simulink model "six_plus_six_AcmsteeringV09_main_1lf"  (R2014a)
settings: Solver=FixedStepDiscrete  StartTime=0.0  StopTime=10.0  FixedStep=0.0005  RelTol=1e-3
InitFcn:
  | Veh_Par_wxt
undefined symbols (not defined in the file or in its folder): acc_spdctl, ag_thr, B, bra_em, bra_pre_gz2, bra_pre_gz34, bra_pre_yd, brakepre_dem_data, brakeTrq_dem_data, bratrq_max, ecucoder_acal, eff_tran, ESP_switch, G, guzhang_lf, guzhang_lm, guzhang_lr, guzhang_rf, guzhang_rm, guzhang_rr, kd1, kd2, ki1, ki2, kp1, kp2, L, myFIS, premax, Radius, RC_switch, s_opt_yi, s_opt_zhuan, s_opt_zhuan_add, s_opt_zhuan_table, spd_map_mot, spd_spdctl, speed_thr_park, TCS_switch, tras_ratio, trq_map_mot, trqmax_yd, trqmax_zx, trqmaxneg, v_gain, v_table, v_thr_park, zhidong_bianmazhi, zhidong_down, zhidong_up, zhidong_youmen, zhuanxiang_bianmazhi, zhuanxiang_down, zhuanxiang_up, zhuanxiang_youmen
libraries: simulink x980, ec5744lib x59, fuzblock x2
(part 8 of 25)

== matlab function six_plus_six_AcmsteeringV09_main_1lf/MainControl/mode_control/center_steer/center_steer/容错控制/MATLAB Function ==
  data: trq_dem_l input; trq_dem_lf output; trq_dem_lm output; trq_dem_r input; trqlim_lf input; trqlim_lm input; trqlim_lr input; trqlim_rf input; trqlim_rm input; trqlim_rr input; guzhang_lf input; guzhang_lm input; guzhang_lr input; guzhang_rf input; guzhang_rm input; guzhang_rr input; trq_dem_lr output; trq_dem_rf output; trq_dem_rm output; trq_dem_rr output; bra_pre_l output; bra_pre_r output; bra_pre_yd input; mode output; bra_dem_l input; bra_dem_r input; brake_dem input
function [trq_dem_lf,trq_dem_lm,trq_dem_lr,trq_dem_rf,trq_dem_rm,trq_dem_rr,bra_pre_l,bra_pre_r,mode] = fcn(trq_dem_l,trq_dem_r,trqlim_lf,trqlim_lm,trqlim_lr,trqlim_rf,trqlim_rm,trqlim_rr,guzhang_lf,guzhang_lm,guzhang_lr,guzhang_rf,guzhang_rm,guzhang_rr,bra_pre_yd,bra_dem_l,bra_dem_r,brake_dem)
%#codegen
if brake_dem==0
    
    trq_dem_lf=single(trq_dem_l/3);
    trq_dem_lm=single(trq_dem_l/3);
    trq_dem_lr=single(trq_dem_l/3);
    trq_dem_rf=single(trq_dem_r/3);
    trq_dem_rm=single(trq_dem_r/3);
    trq_dem_rr=single(trq_dem_r/3);
    bra_pre_l=single(0);
    bra_pre_r=single(0);
    mode=1;
    
    
    %     if guzhang_lf==0 && guzhang_lr==0 && guzhang_rf==0 && guzhang_rr==0    %0电机故障,平均分配
    %         trq_dem_lf=single(trq_dem_l/2);
    %         trq_dem_lr=single(trq_dem_l/2);
    %         trq_dem_rf=single(trq_dem_r/2);
    %         trq_dem_rr=single(trq_dem_r/2);
    %         bra_pre_l=single(0);
    %         bra_pre_r=single(0);
    %         mode=1;
    %     elseif  guzhang_lf==1 && guzhang_lr==0 && guzhang_rf==0 && guzhang_rr==0  %1电机故障，同侧电机进行力矩转移,跟行车不同，对侧不降扭。
    %         trq_dem_lf=single(0);
    %         trq_dem_lr=single(min(trq_dem_l,trqlim_lr));
    %         trq_dem_rf=single(trq_dem_r/2);
    %         trq_dem_rr=single(trq_dem_r/2);
    %         bra_pre_l=single(0);
    %         bra_pre_r=single(0);
    %         mode=2;
    %     elseif  guzhang_lf==0 && guzhang_lr==1 && guzhang_rf==0 && guzhang_rr==0
    %         trq_dem_lf=single(min(trq_dem_l,trqlim_lf));
    %         trq_dem_lr=single(0);
    %         trq_dem_rf=single(trq_dem_r/2);
    %         trq_dem_rr=single(trq_dem_r/2);
    %         bra_pre_l=single(0);
    %         bra_pre_r=single(0);
    %         mode=3;
    %     elseif  guzhang_lf==0 && guzhang_lr==0 && guzhang_rf==1 && guzhang_rr==0
    %         trq_dem_rf=single(0);
    %         trq_dem_rr=single(min(trq_dem_r,trqlim_rr));
    %         trq_dem_lf=single(trq_dem_l/2);
    %         trq_dem_lr=single(trq_dem_l/2);
    %         bra_pre_l=single(0);
    %         bra_pre_r=single(0);
    %         mode=4;
    %     elseif  guzhang_lf==0 && guzhang_lr==0 && guzhang_rf==0 && guzhang_rr==1
    %         trq_dem_rf=single(min(trq_dem_r,trqlim_rf));
    %         trq_dem_rr=single(0);
    %         trq_dem_lf=single(trq_dem_l/2);
    %         trq_dem_lr=single(trq_dem_l/2);
    %         bra_pre_l=single(0);
    %         bra_pre_r=single(0);
    %         mode=5;
    %     elseif  guzhang_lf==1 && guzhang_lr==1 && guzhang_rf==0 && guzhang_rr==0  %2电机故障，左侧双电机故障，左侧履带施加制动，改为原地转向
    %         trq_dem_lf=single(0);
    %         trq_dem_lr=single(0);
    %         trq_dem_rf=single(trq_dem_r/2);
    %         trq_dem_rr=single(trq_dem_r/2);
    %         bra_pre_l=single(bra_pre_yd);
    %         bra_pre_r=single(0);
    %         mode=6;
    %     elseif  guzhang_lf==0 && guzhang_lr==0 && guzhang_rf==1 && guzhang_rr==1  %右侧双电机故障
    %         trq_dem_lf=single(trq_dem_l/2);
    %         trq_dem_lr=single(trq_dem_l/2);
    %         trq_dem_rf=single(0);
    %         trq_dem_rr=single(0);
    %         bra_pre_l=single(0);
    %         bra_pre_r=single(bra_pre_yd);
    %         mode=7;
    %     elseif  guzhang_lf==1 && guzhang_lr==0 && guzhang_rf==1 && guzhang_rr==0 %2电机故障，对侧双电机故障,有4种情况,前两电机故障
    %         trq_dem_lf=single(0);
    %         trq_dem_rf=single(0);
    %         trq_dem_lr=single(min(trq_dem_l,trqlim_lr));
    %         trq_dem_rr=single(min(trq_dem_r,trqlim_rr));
    %         bra_pre_l=single(0);
    %         bra_pre_r=single(0);
    %         mode=8;
    %     elseif  guzhang_lf==0 && guzhang_lr==1 && guzhang_rf==0 && guzhang_rr==1 %后两电机故障
    %         trq_dem_lr=single(0);
    %         trq_dem_rr=single(0);
    %         trq_dem_lf=single(min(trq_dem_l,trqlim_lf));
    %         trq_dem_rf=single(min(trq_dem_r,trqlim_rf));
    %         bra_pre_l=single(0);
    %         bra_pre_r=single(0);
    %         mode=9;
    %     elseif  guzhang_lf==1 && guzhang_lr==0 && guzhang_rf==0 && guzhang_rr==1 %左前电机和右后电机故障
    %         trq_dem_lf=single(0);
    %         trq_dem_rr=single(0);
    %         trq_dem_lr=single(min(trq_dem_l,trqlim_lr));
    %         trq_dem_rf=single(min(trq_dem_r,trqlim_rf));
    %         bra_pre_l=single(0);
    %         bra_pre_r=single(0);
    %         mode=10;
    %     elseif  guzhang_lf==0 && guzhang_lr==1 && guzhang_rf==1 && guzhang_rr==0 %左后电机和右前电机故障
    %         trq_dem_lr=single(0);
    %         trq_dem_rf=single(0);
    %         trq_dem_lf=single(min(trq_dem_l,trqlim_lf));
    %         trq_dem_rr=single(min(trq_dem_r,trqlim_rr));
    %         bra_pre_l=single(0);
    %         bra_pre_r=single(0);
    %         mode=11;
    %     elseif guzhang_lf==1 && guzhang_lr==1 && guzhang_rf==1 && guzhang_rr==0   % 三电机故障
    %         trq_dem_lf=single(0);
    %         trq_dem_lr=single(0);
    %         trq_dem_rf=single(0);
    %         trq_dem_rr=single(min(trq_dem_r,trqlim_rr));
    %         bra_pre_l=single(bra_pre_yd);
    %         bra_pre_r=single(0);
    %         mode=12;
    %     elseif guzhang_lf==1 && guzhang_lr==1 && guzhang_rf==0 && guzhang_rr==1
    %         trq_dem_lf=single(0);
    %         trq_dem_lr=single(0);
    %         trq_dem_rf=single(min(trq_dem_r,trqlim_rf));
    %         trq_dem_rr=single(0);
    %         bra_pre_l=single(bra_pre_yd);
    %         bra_pre_r=single(0);
    %         mode=13;
    %     elseif guzhang_lf==1 && guzhang_lr==0 && guzhang_rf==1 && guzhang_rr==1
    %         trq_dem_lf=single(0);
    %         trq_dem_lr=single(min(trq_dem_l,trqlim_lr));
    %         trq_dem_rf=single(0);
    %         trq_dem_rr=single(0);
    %         bra_pre_l=single(0);
    %         bra_pre_r=single(bra_pre_yd);
    %         mode=14;
    %     elseif guzhang_lf==0 && guzhang_lr==1 && guzhang_rf==1 && guzhang_rr==1
    %         trq_dem_lf=single(min(trq_dem_l,trqlim_lf));
    %         trq_dem_lr=single(0);
    %         trq_dem_rf=single(0);
    %         trq_dem_rr=single(0);
    %         bra_pre_l=single(0);
    %         bra_pre_r=single(bra_pre_yd);
    %         mode=15;
    %     else
    %         %     guzhang_lf==1 && guzhang_lr==1 && guzhang_rf==1 && guzhang_rr==1 %四电机故障
    %         trq_dem_lf=single(0);
    %         trq_dem_lr=single(0);
    %         trq_dem_rf=single(0);
    %         trq_dem_rr=single(0);
    %         bra_pre_l=single(0);
    %         bra_pre_r=single(0);
    %         mode=16;
    %     end
else
    trq_dem_lf=single(0);
    trq_dem_lm=single(0);
    trq_dem_lr=single(0);
    trq_dem_rf=single(0);
    trq_dem_rm=single(0);
    trq_dem_rr=single(0);
    bra_pre_l=single(bra_dem_l);
    bra_pre_r=single(bra_dem_r);
    mode=17;
end
trq_dem_lf=single(min(trqlim_lf,trq_dem_lf));trq_dem_lf=single(max(0,trq_dem_lf));
trq_dem_lm=single(min(trqlim_lm,trq_dem_lm));trq_dem_lm=single(max(0,trq_dem_lm));
trq_dem_lr=single(min(trqlim_lr,trq_dem_lr));trq_dem_lr=single(max(0,trq_dem_lr));
trq_dem_rf=single(min(trqlim_rf,trq_dem_rf));trq_dem_rf=single(max(0,trq_dem_rf));
trq_dem_rm=single(min(trqlim_rm,trq_dem_rm));trq_dem_rm=single(max(0,trq_dem_rm));
trq_dem_rr=single(min(trqlim_rr,trq_dem_rr));trq_dem_rr=single(max(0,trq_dem_rr));
bra_pre_l=single(bra_pre_l);
bra_pre_r=single(bra_pre_r);
end

== system six_plus_six_AcmsteeringV09_main_1lf/Data_input/MCU0_5/MCU0 ==
  input : Inport
  Enable : EnablePort
  Demux : Demux  Outputs=8
  MCU0_ControlMode_Ad : Sum
  MCU0_ControlMode_Convert : DataTypeConversion  OutDataTypeStr=uint32
  MCU0_ControlMode_F : Gain
  MCU0_ControlMode_L : simulink/Logic and Bit Operations/Bitwise Operator  logicop=AND  UseBitMask=on  BitMask=4  BitMaskRealWorld=Stored Integer
  MCU0_ControlMode_O : Constant  Value=0  OutDataTypeStr=single
  MCU0_ControlMode_S : ArithShift  BitShiftNumber=2
  MCU0_ControlMode_Sub : Subsystem
  MCU0_ControlMode_sat : Saturate  UpperLimit=1  LowerLimit=0
  MCU0_ControlModecv : DataTypeConversion
  MCU0_EmergShutDown_Ad : Sum
  MCU0_EmergShutDown_Convert : DataTypeConversion  OutDataTypeStr=uint32
  MCU0_EmergShutDown_F : Gain
  MCU0_EmergShutDown_L : simulink/Logic and Bit Operations/Bitwise Operator  logicop=AND  UseBitMask=on  BitMask=128  BitMaskRealWorld=Stored Integer
  MCU0_EmergShutDown_O : Constant  Value=0  OutDataTypeStr=single
  MCU0_EmergShutDown_S : ArithShift  BitShiftNumber=7
  MCU0_EmergShutDown_Sub : Subsystem
  MCU0_EmergShutDown_sat : Saturate  UpperLimit=1  LowerLimit=0
  MCU0_EmergShutDowncv : DataTypeConversion
  MCU0_GearStatus_Ad : Sum
  MCU0_GearStatus_Convert : DataTypeConversion  OutDataTypeStr=uint32
  MCU0_GearStatus_F : Gain
  MCU0_GearStatus_L : simulink/Logic and Bit Operations/Bitwise Operator  logicop=AND  UseBitMask=on  BitMask=24  BitMaskRealWorld=Stored Integer
  MCU0_GearStatus_O : Constant  Value=0  OutDataTypeStr=single
  MCU0_GearStatus_S : ArithShift  BitShiftNumber=3
  MCU0_GearStatus_Sub : Subsystem
  MCU0_GearStatus_sat : Saturate  UpperLimit=3  LowerLimit=0
  MCU0_GearStatuscv : DataTypeConversion
  MCU0_HighVol_Ad : Sum
  MCU0_HighVol_Convert : DataTypeConversion  OutDataTypeStr=uint32
  MCU0_HighVol_F : Gain
  MCU0_HighVol_L : simulink/Logic and Bit Operations/Bitwise Operator  logicop=AND  UseBitMask=on  BitMask=32  BitMaskRealWorld=Stored Integer
  MCU0_HighVol_O : Constant  Value=0  OutDataTypeStr=single
  MCU0_HighVol_S : ArithShift  BitShiftNumber=5
  MCU0_HighVol_Sub : Subsystem
  MCU0_HighVol_sat : Saturate  UpperLimit=1  LowerLimit=0
  MCU0_HighVolcv : DataTypeConversion
  MCU0_LiftCnt_Ad : Sum
  MCU0_LiftCnt_Convert : DataTypeConversion  OutDataTypeStr=uint32
  MCU0_LiftCnt_F : Gain
  MCU0_LiftCnt_L : simulink/Logic and Bit Operations/Bitwise Operator  logicop=AND  UseBitMask=on  BitMask=255  BitMaskRealWorld=Stored Integer
  MCU0_LiftCnt_O : Constant  Value=0  OutDataTypeStr=single
  MCU0_LiftCnt_S : ArithShift
  MCU0_LiftCnt_Sub : Subsystem
  MCU0_LiftCnt_sat : Saturate  UpperLimit=255  LowerLimit=0
  MCU0_LiftCntcv : DataTypeConversion
  MCU0_ShutDowAllow_Ad : Sum
  MCU0_ShutDowAllow_Convert : DataTypeConversion  OutDataTypeStr=uint32
  MCU0_ShutDowAllow_F : Gain
  MCU0_ShutDowAllow_L : simulink/Logic and Bit Operations/Bitwise Operator  logicop=AND  UseBitMask=on  BitMask=64  BitMaskRealWorld=Stored Integer
  MCU0_ShutDowAllow_O : Constant  Value=0  OutDataTypeStr=single
  MCU0_ShutDowAllow_S : ArithShift  BitShiftNumber=6
  MCU0_ShutDowAllow_Sub : Subsystem
  MCU0_ShutDowAllow_sat : Saturate  UpperLimit=1  LowerLimit=0
  MCU0_ShutDowAllowcv : DataTypeConversion
  MCU0_SpeedFdk_Ad : Sum
  MCU0_SpeedFdk_Convert : DataTypeConversion  OutDataTypeStr=uint32
  MCU0_SpeedFdk_F : Gain
  MCU0_SpeedFdk_L : simulink/Logic and Bit Operations/Bitwise Operator  logicop=AND  UseBitMask=on  BitMask=65535  BitMaskRealWorld=Stored Integer
  MCU0_SpeedFdk_O : Constant  Value=-10000  OutDataTypeStr=single
  MCU0_SpeedFdk_S : ArithShift
  MCU0_SpeedFdk_Sub : Subsystem
  MCU0_SpeedFdk_sat : Saturate  UpperLimit=10000  LowerLimit=-10000
  MCU0_SpeedFdkcv : DataTypeConversion
  MCU0_SpeedFdkinput2_Ad : Sum
  MCU0_SpeedFdkinput2_C : Constant  Value=256
  MCU0_SpeedFdkinput2_P : Product
  MCU0_TorqueFdk_Ad : Sum
  MCU0_TorqueFdk_Convert : DataTypeConversion  OutDataTypeStr=uint32
  MCU0_TorqueFdk_F : Gain  Gain=0.1
  MCU0_TorqueFdk_L : simulink/Logic and Bit Operations/Bitwise Operator  logicop=AND  UseBitMask=on  BitMask=65535  BitMaskRealWorld=Stored Integer
  MCU0_TorqueFdk_O : Constant  Value=-1000  OutDataTypeStr=single
  MCU0_TorqueFdk_S : ArithShift
  MCU0_TorqueFdk_Sub : Subsystem
  MCU0_TorqueFdk_sat : Saturate  UpperLimit=1000  LowerLimit=-1000
  MCU0_TorqueFdkcv : DataTypeConversion
  MCU0_TorqueFdkinput4_Ad : Sum
  MCU0_TorqueFdkinput4_C : Constant  Value=256
  MCU0_TorqueFdkinput4_P : Product
  MCU0_TorqueMax_Ad : Sum
  MCU0_TorqueMax_Convert : DataTypeConversion  OutDataTypeStr=uint32
  MCU0_TorqueMax_F : Gain  Gain=0.1
  MCU0_TorqueMax_L : simulink/Logic and Bit Operations/Bitwise Operator  logicop=AND  UseBitMask=on  BitMask=65535  BitMaskRealWorld=Stored Integer
  MCU0_TorqueMax_O : Constant  Value=-1000  OutDataTypeStr=single
  MCU0_TorqueMax_S : ArithShift
  MCU0_TorqueMax_Sub : Subsystem
  MCU0_TorqueMax_sat : Saturate  UpperLimit=1000  LowerLimit=-1000
  MCU0_TorqueMaxcv : DataTypeConversion
  MCU0_TorqueMaxinput6_Ad : Sum
  MCU0_TorqueMaxinput6_C : Constant  Value=256
  MCU0_TorqueMaxinput6_P : Product
  MCU0_WorkStatus_Ad : Sum
  MCU0_WorkStatus_Convert : DataTypeConversion  OutDataTypeStr=uint32
  MCU0_WorkStatus_F : Gain
  MCU0_WorkStatus_L : simulink/Logic and Bit Operations/Bitwise Operator  logicop=AND  UseBitMask=on  BitMask=3  BitMaskRealWorld=Stored Integer
  MCU0_WorkStatus_O : Constant  Value=0  OutDataTypeStr=single
  MCU0_WorkStatus_S : ArithShift
  MCU0_WorkStatus_Sub : Subsystem
  MCU0_WorkStatus_sat : Saturate  UpperLimit=3  LowerLimit=0
  MCU0_WorkStatuscv : DataTypeConversion
  MCU0_TorqueMax_Out : Outport
  MCU0_EmergShutDown_Out : Outport  Port=2
  MCU0_ShutDowAllow_Out : Outport  Port=3
  MCU0_HighVol_Out : Outport  Port=4
  MCU0_LiftCnt_Out : Outport  Port=5
  MCU0_TorqueFdk_Out : Outport  Port=6
  MCU0_SpeedFdk_Out : Outport  Port=7
  MCU0_GearStatus_Out : Outport  Port=8
  MCU0_ControlMode_Out : Outport  Port=9
  MCU0_WorkStatus_Out : Outport  Port=10
  wires:
  MCU0_TorqueMax_F/1 -> MCU0_TorqueMax_Ad/1
  MCU0_TorqueMax_O/1 -> MCU0_TorqueMax_Ad/2
  MCU0_TorqueMax_Ad/1 -> MCU0_TorqueMax_sat/1
  MCU0_TorqueMax_sat/1 -> MCU0_TorqueMax_Out/1
  Demux/6 -> MCU0_TorqueMaxinput6_P/1
  MCU0_TorqueMaxinput6_C/1 -> MCU0_TorqueMaxinput6_P/2
  MCU0_TorqueMaxinput6_P/1 -> MCU0_TorqueMaxinput6_Ad/1
  Demux/7 -> MCU0_TorqueMaxinput6_Ad/2
  MCU0_TorqueMaxinput6_Ad/1 -> MCU0_TorqueMax_Sub/1(In1)
  MCU0_TorqueMax_Sub/1(Out1) -> MCU0_TorqueMax_Convert/1
  MCU0_TorqueMax_Convert/1 -> MCU0_TorqueMax_L/1
  MCU0_TorqueMax_L/1 -> MCU0_TorqueMax_S/1
  MCU0_TorqueMax_S/1 -> MCU0_TorqueMaxcv/1
  MCU0_TorqueMaxcv/1 -> MCU0_TorqueMax_F/1
  MCU0_EmergShutDown_F/1 -> MCU0_EmergShutDown_Ad/1
  MCU0_EmergShutDown_O/1 -> MCU0_EmergShutDown_Ad/2
  MCU0_EmergShutDown_Ad/1 -> MCU0_EmergShutDown_sat/1
  MCU0_EmergShutDown_sat/1 -> MCU0_EmergShutDown_Out/1
  Demux/1 -> MCU0_ControlMode_Sub/1(In1), MCU0_WorkStatus_Sub/1(In1), MCU0_GearStatus_Sub/1(In1), MCU0_HighVol_Sub/1(In1), MCU0_ShutDowAllow_Sub/1(In1), MCU0_EmergShutDown_Sub/1(In1)
  MCU0_EmergShutDown_Sub/1(Out1) -> MCU0_EmergShutDown_Convert/1
  MCU0_EmergShutDown_Convert/1 -> MCU0_EmergShutDown_L/1
  MCU0_EmergShutDown_L/1 -> MCU0_EmergShutDown_S/1
  MCU0_EmergShutDown_S/1 -> MCU0_EmergShutDowncv/1
  MCU0_EmergShutDowncv/1 -> MCU0_EmergShutDown_F/1
  MCU0_ShutDowAllow_F/1 -> MCU0_ShutDowAllow_Ad/1
  MCU0_ShutDowAllow_O/1 -> MCU0_ShutDowAllow_Ad/2
  MCU0_ShutDowAllow_Ad/1 -> MCU0_ShutDowAllow_sat/1
  MCU0_ShutDowAllow_sat/1 -> MCU0_ShutDowAllow_Out/1
  MCU0_ShutDowAllow_Sub/1(Out1) -> MCU0_ShutDowAllow_Convert/1
  MCU0_ShutDowAllow_Convert/1 -> MCU0_ShutDowAllow_L/1
  MCU0_ShutDowAllow_L/1 -> MCU0_ShutDowAllow_S/1
  MCU0_ShutDowAllow_S/1 -> MCU0_ShutDowAllowcv/1
  MCU0_ShutDowAllowcv/1 -> MCU0_ShutDowAllow_F/1
  MCU0_HighVol_F/1 -> MCU0_HighVol_Ad/1
  MCU0_HighVol_O/1 -> MCU0_HighVol_Ad/2
  MCU0_HighVol_Ad/1 -> MCU0_HighVol_sat/1
  MCU0_HighVol_sat/1 -> MCU0_HighVol_Out/1
  MCU0_HighVol_Sub/1(Out1) -> MCU0_HighVol_Convert/1
  MCU0_HighVol_Convert/1 -> MCU0_HighVol_L/1
  MCU0_HighVol_L/1 -> MCU0_HighVol_S/1
  MCU0_HighVol_S/1 -> MCU0_HighVolcv/1
  MCU0_HighVolcv/1 -> MCU0_HighVol_F/1
  MCU0_LiftCnt_F/1 -> MCU0_LiftCnt_Ad/1
  MCU0_LiftCnt_O/1 -> MCU0_LiftCnt_Ad/2
  MCU0_LiftCnt_Ad/1 -> MCU0_LiftCnt_sat/1
  MCU0_LiftCnt_sat/1 -> MCU0_LiftCnt_Out/1
  Demux/8 -> MCU0_LiftCnt_Sub/1(In1)
  MCU0_LiftCnt_Sub/1(Out1) -> MCU0_LiftCnt_Convert/1
  MCU0_LiftCnt_Convert/1 -> MCU0_LiftCnt_L/1
  MCU0_LiftCnt_L/1 -> MCU0_LiftCnt_S/1
  MCU0_LiftCnt_S/1 -> MCU0_LiftCntcv/1
  MCU0_LiftCntcv/1 -> MCU0_LiftCnt_F/1
  MCU0_TorqueFdk_F/1 -> MCU0_TorqueFdk_Ad/1
  MCU0_TorqueFdk_O/1 -> MCU0_TorqueFdk_Ad/2
  MCU0_TorqueFdk_Ad/1 -> MCU0_TorqueFdk_sat/1
  MCU0_TorqueFdk_sat/1 -> MCU0_TorqueFdk_Out/1
  Demux/4 -> MCU0_TorqueFdkinput4_P/1
  MCU0_TorqueFdkinput4_C/1 -> MCU0_TorqueFdkinput4_P/2
  MCU0_TorqueFdkinput4_P/1 -> MCU0_TorqueFdkinput4_Ad/1
  Demux/5 -> MCU0_TorqueFdkinput4_Ad/2
  MCU0_TorqueFdkinput4_Ad/1 -> MCU0_TorqueFdk_Sub/1(In1)
  MCU0_TorqueFdk_Sub/1(Out1) -> MCU0_TorqueFdk_Convert/1
  MCU0_TorqueFdk_Convert/1 -> MCU0_TorqueFdk_L/1
  MCU0_TorqueFdk_L/1 -> MCU0_TorqueFdk_S/1
  MCU0_TorqueFdk_S/1 -> MCU0_TorqueFdkcv/1
  MCU0_TorqueFdkcv/1 -> MCU0_TorqueFdk_F/1
  MCU0_SpeedFdk_F/1 -> MCU0_SpeedFdk_Ad/1
  MCU0_SpeedFdk_O/1 -> MCU0_SpeedFdk_Ad/2
  MCU0_SpeedFdk_Ad/1 -> MCU0_SpeedFdk_sat/1
  MCU0_SpeedFdk_sat/1 -> MCU0_SpeedFdk_Out/1
  Demux/2 -> MCU0_SpeedFdkinput2_P/1
  MCU0_SpeedFdkinput2_C/1 -> MCU0_SpeedFdkinput2_P/2
  MCU0_SpeedFdkinput2_P/1 -> MCU0_SpeedFdkinput2_Ad/1
  Demux/3 -> MCU0_SpeedFdkinput2_Ad/2
  MCU0_SpeedFdkinput2_Ad/1 -> MCU0_SpeedFdk_Sub/1(In1)
  MCU0_SpeedFdk_Sub/1(Out1) -> MCU0_SpeedFdk_Convert/1
  MCU0_SpeedFdk_Convert/1 -> MCU0_SpeedFdk_L/1
  MCU0_SpeedFdk_L/1 -> MCU0_SpeedFdk_S/1
  MCU0_SpeedFdk_S/1 -> MCU0_SpeedFdkcv/1
  MCU0_SpeedFdkcv/1 -> MCU0_SpeedFdk_F/1
  MCU0_GearStatus_F/1 -> MCU0_GearStatus_Ad/1
  MCU0_GearStatus_O/1 -> MCU0_GearStatus_Ad/2
  MCU0_GearStatus_Ad/1 -> MCU0_GearStatus_sat/1
  MCU0_GearStatus_sat/1 -> MCU0_GearStatus_Out/1
  MCU0_GearStatus_Sub/1(Out1) -> MCU0_GearStatus_Convert/1
  MCU0_GearStatus_Convert/1 -> MCU0_GearStatus_L/1
  MCU0_GearStatus_L/1 -> MCU0_GearStatus_S/1
  MCU0_GearStatus_S/1 -> MCU0_GearStatuscv/1
  MCU0_GearStatuscv/1 -> MCU0_GearStatus_F/1
  MCU0_ControlMode_F/1 -> MCU0_ControlMode_Ad/1
  MCU0_ControlMode_O/1 -> MCU0_ControlMode_Ad/2
  MCU0_ControlMode_Ad/1 -> MCU0_ControlMode_sat/1
  MCU0_ControlMode_sat/1 -> MCU0_ControlMode_Out/1
  MCU0_ControlMode_Sub/1(Out1) -> MCU0_ControlMode_Convert/1
  MCU0_ControlMode_Convert/1 -> MCU0_ControlMode_L/1
  MCU0_ControlMode_L/1 -> MCU0_ControlMode_S/1
  MCU0_ControlMode_S/1 -> MCU0_ControlModecv/1
  MCU0_ControlModecv/1 -> MCU0_ControlMode_F/1
  MCU0_WorkStatus_F/1 -> MCU0_WorkStatus_Ad/1
  MCU0_WorkStatus_O/1 -> MCU0_WorkStatus_Ad/2
  MCU0_WorkStatus_Ad/1 -> MCU0_WorkStatus_sat/1
  MCU0_WorkStatus_sat/1 -> MCU0_WorkStatus_Out/1
  MCU0_WorkStatus_Sub/1(Out1) -> MCU0_WorkStatus_Convert/1
  MCU0_WorkStatus_Convert/1 -> MCU0_WorkStatus_L/1
  MCU0_WorkStatus_L/1 -> MCU0_WorkStatus_S/1
  MCU0_WorkStatus_S/1 -> MCU0_WorkStatuscv/1
  MCU0_WorkStatuscv/1 -> MCU0_WorkStatus_F/1
  input/1 -> Demux/1

== system six_plus_six_AcmsteeringV09_main_1lf/Data_input/MCU1/MCU1 ==
  input : Inport
  Enable : EnablePort
  Demux : Demux  Outputs=8
  MCU1_ControlTemp_Ad : Sum
  MCU1_ControlTemp_Convert : DataTypeConversion  OutDataTypeStr=uint32
  MCU1_ControlTemp_F : Gain
  MCU1_ControlTemp_L : simulink/Logic and Bit Operations/Bitwise Operator  logicop=AND  UseBitMask=on  BitMask=255  BitMaskRealWorld=Stored Integer
  MCU1_ControlTemp_O : Constant  Value=-40  OutDataTypeStr=single
  MCU1_ControlTemp_S : ArithShift
  MCU1_ControlTemp_Sub : Subsystem
  MCU1_ControlTemp_sat : Saturate  UpperLimit=215  LowerLimit=-40
  MCU1_ControlTempcv : DataTypeConversion
  MCU1_Idc_Ad : Sum
  MCU1_Idc_Convert : DataTypeConversion  OutDataTypeStr=uint32
  MCU1_Idc_F : Gain  Gain=0.1
  MCU1_Idc_L : simulink/Logic and Bit Operations/Bitwise Operator  logicop=AND  UseBitMask=on  BitMask=65535  BitMaskRealWorld=Stored Integer
  MCU1_Idc_O : Constant  Value=-1600  OutDataTypeStr=single
  MCU1_Idc_S : ArithShift
  MCU1_Idc_Sub : Subsystem
  MCU1_Idc_sat : Saturate  UpperLimit=1600  LowerLimit=-1600
  MCU1_Idccv : DataTypeConversion
  MCU1_Idcinput3_Ad : Sum
  MCU1_Idcinput3_C : Constant  Value=256
  MCU1_Idcinput3_P : Product
  MCU1_MotorTemp_Ad : Sum
  MCU1_MotorTemp_Convert : DataTypeConversion  OutDataTypeStr=uint32
  MCU1_MotorTemp_F : Gain
  MCU1_MotorTemp_L : simulink/Logic and Bit Operations/Bitwise Operator  logicop=AND  UseBitMask=on  BitMask=255  BitMaskRealWorld=Stored Integer
  MCU1_MotorTemp_O : Constant  Value=-40  OutDataTypeStr=single
  MCU1_MotorTemp_S : ArithShift
  MCU1_MotorTemp_Sub : Subsystem
  MCU1_MotorTemp_sat : Saturate  UpperLimit=215  LowerLimit=-40
  MCU1_MotorTempcv : DataTypeConversion
  MCU1_PowerFdk_Ad : Sum
  MCU1_PowerFdk_Convert : DataTypeConversion  OutDataTypeStr=uint32
  MCU1_PowerFdk_F : Gain
  MCU1_PowerFdk_L : simulink/Logic and Bit Operations/Bitwise Operator  logicop=AND  UseBitMask=on  BitMask=65535  BitMaskRealWorld=Stored Integer
  MCU1_PowerFdk_O : Constant  Value=0  OutDataTypeStr=single
  MCU1_PowerFdk_S : ArithShift
  MCU1_PowerFdk_Sub : Subsystem
  MCU1_PowerFdk_sat : Saturate  UpperLimit=65535  LowerLimit=0
  MCU1_PowerFdkcv : DataTypeConversion
  MCU1_PowerFdkinput5_Ad : Sum
  MCU1_PowerFdkinput5_C : Constant  Value=256
  MCU1_PowerFdkinput5_P : Product
  MCU1_Udc_Ad : Sum
  MCU1_Udc_Convert : DataTypeConversion  OutDataTypeStr=uint32
  MCU1_Udc_F : Gain  Gain=0.1
  MCU1_Udc_L : simulink/Logic and Bit Operations/Bitwise Operator  logicop=AND  UseBitMask=on  BitMask=65535  BitMaskRealWorld=Stored Integer
  MCU1_Udc_O : Constant  Value=0  OutDataTypeStr=single
  MCU1_Udc_S : ArithShift
  MCU1_Udc_Sub : Subsystem
  MCU1_Udc_sat : Saturate  UpperLimit=1000  LowerLimit=0
  MCU1_Udccv : DataTypeConversion
  MCU1_Udcinput1_Ad : Sum
  MCU1_Udcinput1_C : Constant  Value=256
  MCU1_Udcinput1_P : Product
  MCU1_ControlTemp_Out : Outport
  MCU1_MotorTemp_Out : Outport  Port=2
  MCU1_PowerFdk_Out : Outport  Port=3
  MCU1_Idc_Out : Outport  Port=4
  MCU1_Udc_Out : Outport  Port=5
  wires:
  MCU1_ControlTemp_F/1 -> MCU1_ControlTemp_Ad/1
  MCU1_ControlTemp_O/1 -> MCU1_ControlTemp_Ad/2
  MCU1_ControlTemp_Ad/1 -> MCU1_ControlTemp_sat/1
  MCU1_ControlTemp_sat/1 -> MCU1_ControlTemp_Out/1
  Demux/8 -> MCU1_ControlTemp_Sub/1(In1)
  MCU1_ControlTemp_Sub/1(Out1) -> MCU1_ControlTemp_Convert/1
  MCU1_ControlTemp_Convert/1 -> MCU1_ControlTemp_L/1
  MCU1_ControlTemp_L/1 -> MCU1_ControlTemp_S/1
  MCU1_ControlTemp_S/1 -> MCU1_ControlTempcv/1
  MCU1_ControlTempcv/1 -> MCU1_ControlTemp_F/1
  MCU1_MotorTemp_F/1 -> MCU1_MotorTemp_Ad/1
  MCU1_MotorTemp_O/1 -> MCU1_MotorTemp_Ad/2
  MCU1_MotorTemp_Ad/1 -> MCU1_MotorTemp_sat/1
  MCU1_MotorTemp_sat/1 -> MCU1_MotorTemp_Out/1
  Demux/7 -> MCU1_MotorTemp_Sub/1(In1)
  MCU1_MotorTemp_Sub/1(Out1) -> MCU1_MotorTemp_Convert/1
  MCU1_MotorTemp_Convert/1 -> MCU1_MotorTemp_L/1
  MCU1_MotorTemp_L/1 -> MCU1_MotorTemp_S/1
  MCU1_MotorTemp_S/1 -> MCU1_MotorTempcv/1
  MCU1_MotorTempcv/1 -> MCU1_MotorTemp_F/1
  MCU1_PowerFdk_F/1 -> MCU1_PowerFdk_Ad/1
  MCU1_PowerFdk_O/1 -> MCU1_PowerFdk_Ad/2
  MCU1_PowerFdk_Ad/1 -> MCU1_PowerFdk_sat/1
  MCU1_PowerFdk_sat/1 -> MCU1_PowerFdk_Out/1
  Demux/5 -> MCU1_PowerFdkinput5_P/1
  MCU1_PowerFdkinput5_C/1 -> MCU1_PowerFdkinput5_P/2
  MCU1_PowerFdkinput5_P/1 -> MCU1_PowerFdkinput5_Ad/1
  Demux/6 -> MCU1_PowerFdkinput5_Ad/2
  MCU1_PowerFdkinput5_Ad/1 -> MCU1_PowerFdk_Sub/1(In1)
  MCU1_PowerFdk_Sub/1(Out1) -> MCU1_PowerFdk_Convert/1
  MCU1_PowerFdk_Convert/1 -> MCU1_PowerFdk_L/1
  MCU1_PowerFdk_L/1 -> MCU1_PowerFdk_S/1
  MCU1_PowerFdk_S/1 -> MCU1_PowerFdkcv/1
  MCU1_PowerFdkcv/1 -> MCU1_PowerFdk_F/1
  MCU1_Idc_F/1 -> MCU1_Idc_Ad/1
  MCU1_Idc_O/1 -> MCU1_Idc_Ad/2
  MCU1_Idc_Ad/1 -> MCU1_Idc_sat/1
  MCU1_Idc_sat/1 -> MCU1_Idc_Out/1
  Demux/3 -> MCU1_Idcinput3_P/1
  MCU1_Idcinput3_C/1 -> MCU1_Idcinput3_P/2
  MCU1_Idcinput3_P/1 -> MCU1_Idcinput3_Ad/1
  Demux/4 -> MCU1_Idcinput3_Ad/2
  MCU1_Idcinput3_Ad/1 -> MCU1_Idc_Sub/1(In1)
  MCU1_Idc_Sub/1(Out1) -> MCU1_Idc_Convert/1
  MCU1_Idc_Convert/1 -> MCU1_Idc_L/1
  MCU1_Idc_L/1 -> MCU1_Idc_S/1
  MCU1_Idc_S/1 -> MCU1_Idccv/1
  MCU1_Idccv/1 -> MCU1_Idc_F/1
  MCU1_Udc_F/1 -> MCU1_Udc_Ad/1
  MCU1_Udc_O/1 -> MCU1_Udc_Ad/2
  MCU1_Udc_Ad/1 -> MCU1_Udc_sat/1
  MCU1_Udc_sat/1 -> MCU1_Udc_Out/1
  Demux/1 -> MCU1_Udcinput1_P/1
  MCU1_Udcinput1_C/1 -> MCU1_Udcinput1_P/2
  MCU1_Udcinput1_P/1 -> MCU1_Udcinput1_Ad/1
  Demux/2 -> MCU1_Udcinput1_Ad/2
  MCU1_Udcinput1_Ad/1 -> MCU1_Udc_Sub/1(In1)
  MCU1_Udc_Sub/1(Out1) -> MCU1_Udc_Convert/1
  MCU1_Udc_Convert/1 -> MCU1_Udc_L/1
  MCU1_Udc_L/1 -> MCU1_Udc_S/1
  MCU1_Udc_S/1 -> MCU1_Udccv/1
  MCU1_Udccv/1 -> MCU1_Udc_F/1
  input/1 -> Demux/1

== system six_plus_six_AcmsteeringV09_main_1lf/Data_input/MCU1_1/MCU1 ==
  input : Inport
  Enable : EnablePort
  Demux : Demux  Outputs=8
  MCU1_ControlTemp_Ad : Sum
  MCU1_ControlTemp_Convert : DataTypeConversion  OutDataTypeStr=uint32
  MCU1_ControlTemp_F : Gain
  MCU1_ControlTemp_L : simulink/Logic and Bit Operations/Bitwise Operator  logicop=AND  UseBitMask=on  BitMask=255  BitMaskRealWorld=Stored Integer
  MCU1_ControlTemp_O : Constant  Value=-40  OutDataTypeStr=single
  MCU1_ControlTemp_S : ArithShift
  MCU1_ControlTemp_Sub : Subsystem
  MCU1_ControlTemp_sat : Saturate  UpperLimit=215  LowerLimit=-40
  MCU1_ControlTempcv : DataTypeConversion
  MCU1_Idc_Ad : Sum
  MCU1_Idc_Convert : DataTypeConversion  OutDataTypeStr=uint32
  MCU1_Idc_F : Gain  Gain=0.1
  MCU1_Idc_L : simulink/Logic and Bit Operations/Bitwise Operator  logicop=AND  UseBitMask=on  BitMask=65535  BitMaskRealWorld=Stored Integer
  MCU1_Idc_O : Constant  Value=-1600  OutDataTypeStr=single
  MCU1_Idc_S : ArithShift
  MCU1_Idc_Sub : Subsystem
  MCU1_Idc_sat : Saturate  UpperLimit=1600  LowerLimit=-1600
  MCU1_Idccv : DataTypeConversion
  MCU1_Idcinput3_Ad : Sum
  MCU1_Idcinput3_C : Constant  Value=256
  MCU1_Idcinput3_P : Product
  MCU1_MotorTemp_Ad : Sum
  MCU1_MotorTemp_Convert : DataTypeConversion  OutDataTypeStr=uint32
  MCU1_MotorTemp_F : Gain
  MCU1_MotorTemp_L : simulink/Logic and Bit Operations/Bitwise Operator  logicop=AND  UseBitMask=on  BitMask=255  BitMaskRealWorld=Stored Integer
  MCU1_MotorTemp_O : Constant  Value=-40  OutDataTypeStr=single
  MCU1_MotorTemp_S : ArithShift
  MCU1_MotorTemp_Sub : Subsystem
  MCU1_MotorTemp_sat : Saturate  UpperLimit=215  LowerLimit=-40
  MCU1_MotorTempcv : DataTypeConversion
  MCU1_PowerFdk_Ad : Sum
  MCU1_PowerFdk_Convert : DataTypeConversion  OutDataTypeStr=uint32
  MCU1_PowerFdk_F : Gain
  MCU1_PowerFdk_L : simulink/Logic and Bit Operations/Bitwise Operator  logicop=AND  UseBitMask=on  BitMask=65535  BitMaskRealWorld=Stored Integer
  MCU1_PowerFdk_O : Constant  Value=0  OutDataTypeStr=single
  MCU1_PowerFdk_S : ArithShift
  MCU1_PowerFdk_Sub : Subsystem
  MCU1_PowerFdk_sat : Saturate  UpperLimit=65535  LowerLimit=0
  MCU1_PowerFdkcv : DataTypeConversion
  MCU1_PowerFdkinput5_Ad : Sum
  MCU1_PowerFdkinput5_C : Constant  Value=256
  MCU1_PowerFdkinput5_P : Product
  MCU1_Udc_Ad : Sum
  MCU1_Udc_Convert : DataTypeConversion  OutDataTypeStr=uint32
  MCU1_Udc_F : Gain  Gain=0.1
  MCU1_Udc_L : simulink/Logic and Bit Operations/Bitwise Operator  logicop=AND  UseBitMask=on  BitMask=65535  BitMaskRealWorld=Stored Integer
  MCU1_Udc_O : Constant  Value=0  OutDataTypeStr=single
  MCU1_Udc_S : ArithShift
  MCU1_Udc_Sub : Subsystem
  MCU1_Udc_sat : Saturate  UpperLimit=1000  LowerLimit=0
  MCU1_Udccv : DataTypeConversion
  MCU1_Udcinput1_Ad : Sum
  MCU1_Udcinput1_C : Constant  Value=256
  MCU1_Udcinput1_P : Product
  MCU1_ControlTemp_Out : Outport
  MCU1_MotorTemp_Out : Outport  Port=2
  MCU1_PowerFdk_Out : Outport  Port=3
  MCU1_Idc_Out : Outport  Port=4
  MCU1_Udc_Out : Outport  Port=5
  wires:
  MCU1_ControlTemp_F/1 -> MCU1_ControlTemp_Ad/1
  MCU1_ControlTemp_O/1 -> MCU1_ControlTemp_Ad/2
  MCU1_ControlTemp_Ad/1 -> MCU1_ControlTemp_sat/1
  MCU1_ControlTemp_sat/1 -> MCU1_ControlTemp_Out/1
  Demux/8 -> MCU1_ControlTemp_Sub/1(In1)
  MCU1_ControlTemp_Sub/1(Out1) -> MCU1_ControlTemp_Convert/1
  MCU1_ControlTemp_Convert/1 -> MCU1_ControlTemp_L/1
  MCU1_ControlTemp_L/1 -> MCU1_ControlTemp_S/1
  MCU1_ControlTemp_S/1 -> MCU1_ControlTempcv/1
  MCU1_ControlTempcv/1 -> MCU1_ControlTemp_F/1
  MCU1_MotorTemp_F/1 -> MCU1_MotorTemp_Ad/1
  MCU1_MotorTemp_O/1 -> MCU1_MotorTemp_Ad/2
  MCU1_MotorTemp_Ad/1 -> MCU1_MotorTemp_sat/1
  MCU1_MotorTemp_sat/1 -> MCU1_MotorTemp_Out/1
  Demux/7 -> MCU1_MotorTemp_Sub/1(In1)
  MCU1_MotorTemp_Sub/1(Out1) -> MCU1_MotorTemp_Convert/1
  MCU1_MotorTemp_Convert/1 -> MCU1_MotorTemp_L/1
  MCU1_MotorTemp_L/1 -> MCU1_MotorTemp_S/1
  MCU1_MotorTemp_S/1 -> MCU1_MotorTempcv/1
  MCU1_MotorTempcv/1 -> MCU1_MotorTemp_F/1
  MCU1_PowerFdk_F/1 -> MCU1_PowerFdk_Ad/1
  MCU1_PowerFdk_O/1 -> MCU1_PowerFdk_Ad/2
  MCU1_PowerFdk_Ad/1 -> MCU1_PowerFdk_sat/1
  MCU1_PowerFdk_sat/1 -> MCU1_PowerFdk_Out/1
  Demux/5 -> MCU1_PowerFdkinput5_P/1
  MCU1_PowerFdkinput5_C/1 -> MCU1_PowerFdkinput5_P/2
  MCU1_PowerFdkinput5_P/1 -> MCU1_PowerFdkinput5_Ad/1
  Demux/6 -> MCU1_PowerFdkinput5_Ad/2
  MCU1_PowerFdkinput5_Ad/1 -> MCU1_PowerFdk_Sub/1(In1)
  MCU1_PowerFdk_Sub/1(Out1) -> MCU1_PowerFdk_Convert/1
  MCU1_PowerFdk_Convert/1 -> MCU1_PowerFdk_L/1
  MCU1_PowerFdk_L/1 -> MCU1_PowerFdk_S/1
  MCU1_PowerFdk_S/1 -> MCU1_PowerFdkcv/1
  MCU1_PowerFdkcv/1 -> MCU1_PowerFdk_F/1
  MCU1_Idc_F/1 -> MCU1_Idc_Ad/1
  MCU1_Idc_O/1 -> MCU1_Idc_Ad/2
  MCU1_Idc_Ad/1 -> MCU1_Idc_sat/1
  MCU1_Idc_sat/1 -> MCU1_Idc_Out/1
  Demux/3 -> MCU1_Idcinput3_P/1
  MCU1_Idcinput3_C/1 -> MCU1_Idcinput3_P/2
  MCU1_Idcinput3_P/1 -> MCU1_Idcinput3_Ad/1
  Demux/4 -> MCU1_Idcinput3_Ad/2
  MCU1_Idcinput3_Ad/1 -> MCU1_Idc_Sub/1(In1)
  MCU1_Idc_Sub/1(Out1) -> MCU1_Idc_Convert/1
  MCU1_Idc_Convert/1 -> MCU1_Idc_L/1
  MCU1_Idc_L/1 -> MCU1_Idc_S/1
  MCU1_Idc_S/1 -> MCU1_Idccv/1
  MCU1_Idccv/1 -> MCU1_Idc_F/1
  MCU1_Udc_F/1 -> MCU1_Udc_Ad/1
  MCU1_Udc_O/1 -> MCU1_Udc_Ad/2
  MCU1_Udc_Ad/1 -> MCU1_Udc_sat/1
  MCU1_Udc_sat/1 -> MCU1_Udc_Out/1
  Demux/1 -> MCU1_Udcinput1_P/1
  MCU1_Udcinput1_C/1 -> MCU1_Udcinput1_P/2
  MCU1_Udcinput1_P/1 -> MCU1_Udcinput1_Ad/1
  Demux/2 -> MCU1_Udcinput1_Ad/2
  MCU1_Udcinput1_Ad/1 -> MCU1_Udc_Sub/1(In1)
  MCU1_Udc_Sub/1(Out1) -> MCU1_Udc_Convert/1
  MCU1_Udc_Convert/1 -> MCU1_Udc_L/1
  MCU1_Udc_L/1 -> MCU1_Udc_S/1
  MCU1_Udc_S/1 -> MCU1_Udccv/1
  MCU1_Udccv/1 -> MCU1_Udc_F/1
  input/1 -> Demux/1

== system six_plus_six_AcmsteeringV09_main_1lf/Data_input/MCU1_2/MCU1 ==
  input : Inport
  Enable : EnablePort
  Demux : Demux  Outputs=8
  MCU1_ControlTemp_Ad : Sum
  MCU1_ControlTemp_Convert : DataTypeConversion  OutDataTypeStr=uint32
  MCU1_ControlTemp_F : Gain
  MCU1_ControlTemp_L : simulink/Logic and Bit Operations/Bitwise Operator  logicop=AND  UseBitMask=on  BitMask=255  BitMaskRealWorld=Stored Integer
  MCU1_ControlTemp_O : Constant  Value=-40  OutDataTypeStr=single
  MCU1_ControlTemp_S : ArithShift
  MCU1_ControlTemp_Sub : Subsystem
  MCU1_ControlTemp_sat : Saturate  UpperLimit=215  LowerLimit=-40
  MCU1_ControlTempcv : DataTypeConversion
  MCU1_Idc_Ad : Sum
  MCU1_Idc_Convert : DataTypeConversion  OutDataTypeStr=uint32
  MCU1_Idc_F : Gain  Gain=0.1
  MCU1_Idc_L : simulink/Logic and Bit Operations/Bitwise Operator  logicop=AND  UseBitMask=on  BitMask=65535  BitMaskRealWorld=Stored Integer
  MCU1_Idc_O : Constant  Value=-1600  OutDataTypeStr=single
  MCU1_Idc_S : ArithShift
  MCU1_Idc_Sub : Subsystem
  MCU1_Idc_sat : Saturate  UpperLimit=1600  LowerLimit=-1600
  MCU1_Idccv : DataTypeConversion
  MCU1_Idcinput3_Ad : Sum
  MCU1_Idcinput3_C : Constant  Value=256
  MCU1_Idcinput3_P : Product
  MCU1_MotorTemp_Ad : Sum
  MCU1_MotorTemp_Convert : DataTypeConversion  OutDataTypeStr=uint32
  MCU1_MotorTemp_F : Gain
  MCU1_MotorTemp_L : simulink/Logic and Bit Operations/Bitwise Operator  logicop=AND  UseBitMask=on  BitMask=255  BitMaskRealWorld=Stored Integer
  MCU1_MotorTemp_O : Constant  Value=-40  OutDataTypeStr=single
  MCU1_MotorTemp_S : ArithShift
  MCU1_MotorTemp_Sub : Subsystem
  MCU1_MotorTemp_sat : Saturate  UpperLimit=215  LowerLimit=-40
  MCU1_MotorTempcv : DataTypeConversion
  MCU1_PowerFdk_Ad : Sum
  MCU1_PowerFdk_Convert : DataTypeConversion  OutDataTypeStr=uint32
  MCU1_PowerFdk_F : Gain
  MCU1_PowerFdk_L : simulink/Logic and Bit Operations/Bitwise Operator  logicop=AND  UseBitMask=on  BitMask=65535  BitMaskRealWorld=Stored Integer
  MCU1_PowerFdk_O : Constant  Value=0  OutDataTypeStr=single
  MCU1_PowerFdk_S : ArithShift
  MCU1_PowerFdk_Sub : Subsystem
  MCU1_PowerFdk_sat : Saturate  UpperLimit=65535  LowerLimit=0
  MCU1_PowerFdkcv : DataTypeConversion
  MCU1_PowerFdkinput5_Ad : Sum
  MCU1_PowerFdkinput5_C : Constant  Value=256
  MCU1_PowerFdkinput5_P : Product
  MCU1_Udc_Ad : Sum
  MCU1_Udc_Convert : DataTypeConversion  OutDataTypeStr=uint32
  MCU1_Udc_F : Gain  Gain=0.1
  MCU1_Udc_L : simulink/Logic and Bit Operations/Bitwise Operator  logicop=AND  UseBitMask=on  BitMask=65535  BitMaskRealWorld=Stored Integer
  MCU1_Udc_O : Constant  Value=0  OutDataTypeStr=single
  MCU1_Udc_S : ArithShift
  MCU1_Udc_Sub : Subsystem
  MCU1_Udc_sat : Saturate  UpperLimit=1000  LowerLimit=0
  MCU1_Udccv : DataTypeConversion
  MCU1_Udcinput1_Ad : Sum
  MCU1_Udcinput1_C : Constant  Value=256
  MCU1_Udcinput1_P : Product
  MCU1_ControlTemp_Out : Outport
  MCU1_MotorTemp_Out : Outport  Port=2
  MCU1_PowerFdk_Out : Outport  Port=3
  MCU1_Idc_Out : Outport  Port=4
  MCU1_Udc_Out : Outport  Port=5
  wires:
  MCU1_ControlTemp_F/1 -> MCU1_ControlTemp_Ad/1
  MCU1_ControlTemp_O/1 -> MCU1_ControlTemp_Ad/2
  MCU1_ControlTemp_Ad/1 -> MCU1_ControlTemp_sat/1
  MCU1_ControlTemp_sat/1 -> MCU1_ControlTemp_Out/1
  Demux/8 -> MCU1_ControlTemp_Sub/1(In1)
  MCU1_ControlTemp_Sub/1(Out1) -> MCU1_ControlTemp_Convert/1
  MCU1_ControlTemp_Convert/1 -> MCU1_ControlTemp_L/1
  MCU1_ControlTemp_L/1 -> MCU1_ControlTemp_S/1
  MCU1_ControlTemp_S/1 -> MCU1_ControlTempcv/1
  MCU1_ControlTempcv/1 -> MCU1_ControlTemp_F/1
  MCU1_MotorTemp_F/1 -> MCU1_MotorTemp_Ad/1
  MCU1_MotorTemp_O/1 -> MCU1_MotorTemp_Ad/2
  MCU1_MotorTemp_Ad/1 -> MCU1_MotorTemp_sat/1
  MCU1_MotorTemp_sat/1 -> MCU1_MotorTemp_Out/1
  Demux/7 -> MCU1_MotorTemp_Sub/1(In1)
  MCU1_MotorTemp_Sub/1(Out1) -> MCU1_MotorTemp_Convert/1
  MCU1_MotorTemp_Convert/1 -> MCU1_MotorTemp_L/1
  MCU1_MotorTemp_L/1 -> MCU1_MotorTemp_S/1
  MCU1_MotorTemp_S/1 -> MCU1_MotorTempcv/1
  MCU1_MotorTempcv/1 -> MCU1_MotorTemp_F/1
  MCU1_PowerFdk_F/1 -> MCU1_PowerFdk_Ad/1
  MCU1_PowerFdk_O/1 -> MCU1_PowerFdk_Ad/2
  MCU1_PowerFdk_Ad/1 -> MCU1_PowerFdk_sat/1
  MCU1_PowerFdk_sat/1 -> MCU1_PowerFdk_Out/1
  Demux/5 -> MCU1_PowerFdkinput5_P/1
  MCU1_PowerFdkinput5_C/1 -> MCU1_PowerFdkinput5_P/2
  MCU1_PowerFdkinput5_P/1 -> MCU1_PowerFdkinput5_Ad/1
  Demux/6 -> MCU1_PowerFdkinput5_Ad/2
  MCU1_PowerFdkinput5_Ad/1 -> MCU1_PowerFdk_Sub/1(In1)
  MCU1_PowerFdk_Sub/1(Out1) -> MCU1_PowerFdk_Convert/1
  MCU1_PowerFdk_Convert/1 -> MCU1_PowerFdk_L/1
  MCU1_PowerFdk_L/1 -> MCU1_PowerFdk_S/1
  MCU1_PowerFdk_S/1 -> MCU1_PowerFdkcv/1
  MCU1_PowerFdkcv/1 -> MCU1_PowerFdk_F/1
  MCU1_Idc_F/1 -> MCU1_Idc_Ad/1
  MCU1_Idc_O/1 -> MCU1_Idc_Ad/2
  MCU1_Idc_Ad/1 -> MCU1_Idc_sat/1
  MCU1_Idc_sat/1 -> MCU1_Idc_Out/1
  Demux/3 -> MCU1_Idcinput3_P/1
  MCU1_Idcinput3_C/1 -> MCU1_Idcinput3_P/2
  MCU1_Idcinput3_P/1 -> MCU1_Idcinput3_Ad/1
  Demux/4 -> MCU1_Idcinput3_Ad/2
  MCU1_Idcinput3_Ad/1 -> MCU1_Idc_Sub/1(In1)
  MCU1_Idc_Sub/1(Out1) -> MCU1_Idc_Convert/1
  MCU1_Idc_Convert/1 -> MCU1_Idc_L/1
  MCU1_Idc_L/1 -> MCU1_Idc_S/1
  MCU1_Idc_S/1 -> MCU1_Idccv/1
  MCU1_Idccv/1 -> MCU1_Idc_F/1
  MCU1_Udc_F/1 -> MCU1_Udc_Ad/1
  MCU1_Udc_O/1 -> MCU1_Udc_Ad/2
  MCU1_Udc_Ad/1 -> MCU1_Udc_sat/1
  MCU1_Udc_sat/1 -> MCU1_Udc_Out/1
  Demux/1 -> MCU1_Udcinput1_P/1
  MCU1_Udcinput1_C/1 -> MCU1_Udcinput1_P/2
  MCU1_Udcinput1_P/1 -> MCU1_Udcinput1_Ad/1
  Demux/2 -> MCU1_Udcinput1_Ad/2
  MCU1_Udcinput1_Ad/1 -> MCU1_Udc_Sub/1(In1)
  MCU1_Udc_Sub/1(Out1) -> MCU1_Udc_Convert/1
  MCU1_Udc_Convert/1 -> MCU1_Udc_L/1
  MCU1_Udc_L/1 -> MCU1_Udc_S/1
  MCU1_Udc_S/1 -> MCU1_Udccv/1
  MCU1_Udccv/1 -> MCU1_Udc_F/1
  input/1 -> Demux/1

== system six_plus_six_AcmsteeringV09_main_1lf/Data_input/MCU1_3/MCU1 ==
  input : Inport
  Enable : EnablePort
  Demux : Demux  Outputs=8
  MCU1_ControlTemp_Ad : Sum
  MCU1_ControlTemp_Convert : DataTypeConversion  OutDataTypeStr=uint32
  MCU1_ControlTemp_F : Gain
  MCU1_ControlTemp_L : simulink/Logic and Bit Operations/Bitwise Operator  logicop=AND  UseBitMask=on  BitMask=255  BitMaskRealWorld=Stored Integer
  MCU1_ControlTemp_O : Constant  Value=-40  OutDataTypeStr=single
  MCU1_ControlTemp_S : ArithShift
  MCU1_ControlTemp_Sub : Subsystem
  MCU1_ControlTemp_sat : Saturate  UpperLimit=215  LowerLimit=-40
  MCU1_ControlTempcv : DataTypeConversion
  MCU1_Idc_Ad : Sum
  MCU1_Idc_Convert : DataTypeConversion  OutDataTypeStr=uint32
  MCU1_Idc_F : Gain  Gain=0.1
  MCU1_Idc_L : simulink/Logic and Bit Operations/Bitwise Operator  logicop=AND  UseBitMask=on  BitMask=65535  BitMaskRealWorld=Stored Integer
  MCU1_Idc_O : Constant  Value=-1600  OutDataTypeStr=single
  MCU1_Idc_S : ArithShift
  MCU1_Idc_Sub : Subsystem
  MCU1_Idc_sat : Saturate  UpperLimit=1600  LowerLimit=-1600
  MCU1_Idccv : DataTypeConversion
  MCU1_Idcinput3_Ad : Sum
  MCU1_Idcinput3_C : Constant  Value=256
  MCU1_Idcinput3_P : Product
  MCU1_MotorTemp_Ad : Sum
  MCU1_MotorTemp_Convert : DataTypeConversion  OutDataTypeStr=uint32
  MCU1_MotorTemp_F : Gain
  MCU1_MotorTemp_L : simulink/Logic and Bit Operations/Bitwise Operator  logicop=AND  UseBitMask=on  BitMask=255  BitMaskRealWorld=Stored Integer
  MCU1_MotorTemp_O : Constant  Value=-40  OutDataTypeStr=single
  MCU1_MotorTemp_S : ArithShift
  MCU1_MotorTemp_Sub : Subsystem
  MCU1_MotorTemp_sat : Saturate  UpperLimit=215  LowerLimit=-40
  MCU1_MotorTempcv : DataTypeConversion
  MCU1_PowerFdk_Ad : Sum
  MCU1_PowerFdk_Convert : DataTypeConversion  OutDataTypeStr=uint32
  MCU1_PowerFdk_F : Gain
  MCU1_PowerFdk_L : simulink/Logic and Bit Operations/Bitwise Operator  logicop=AND  UseBitMask=on  BitMask=65535  BitMaskRealWorld=Stored Integer
  MCU1_PowerFdk_O : Constant  Value=0  OutDataTypeStr=single
  MCU1_PowerFdk_S : ArithShift
  MCU1_PowerFdk_Sub : Subsystem
  MCU1_PowerFdk_sat : Saturate  UpperLimit=65535  LowerLimit=0
  MCU1_PowerFdkcv : DataTypeConversion
  MCU1_PowerFdkinput5_Ad : Sum
  MCU1_PowerFdkinput5_C : Constant  Value=256
  MCU1_PowerFdkinput5_P : Product
  MCU1_Udc_Ad : Sum
  MCU1_Udc_Convert : DataTypeConversion  OutDataTypeStr=uint32
  MCU1_Udc_F : Gain  Gain=0.1
  MCU1_Udc_L : simulink/Logic and Bit Operations/Bitwise Operator  logicop=AND  UseBitMask=on  BitMask=65535  BitMaskRealWorld=Stored Integer
  MCU1_Udc_O : Constant  Value=0  OutDataTypeStr=single
  MCU1_Udc_S : ArithShift
  MCU1_Udc_Sub : Subsystem
  MCU1_Udc_sat : Saturate  UpperLimit=1000  LowerLimit=0
  MCU1_Udccv : DataTypeConversion
  MCU1_Udcinput1_Ad : Sum
  MCU1_Udcinput1_C : Constant  Value=256
  MCU1_Udcinput1_P : Product
  MCU1_ControlTemp_Out : Outport
  MCU1_MotorTemp_Out : Outport  Port=2
  MCU1_PowerFdk_Out : Outport  Port=3
  MCU1_Idc_Out : Outport  Port=4
  MCU1_Udc_Out : Outport  Port=5
  wires:
  MCU1_ControlTemp_F/1 -> MCU1_ControlTemp_Ad/1
  MCU1_ControlTemp_O/1 -> MCU1_ControlTemp_Ad/2
  MCU1_ControlTemp_Ad/1 -> MCU1_ControlTemp_sat/1
  MCU1_ControlTemp_sat/1 -> MCU1_ControlTemp_Out/1
  Demux/8 -> MCU1_ControlTemp_Sub/1(In1)
  MCU1_ControlTemp_Sub/1(Out1) -> MCU1_ControlTemp_Convert/1
  MCU1_ControlTemp_Convert/1 -> MCU1_ControlTemp_L/1
  MCU1_ControlTemp_L/1 -> MCU1_ControlTemp_S/1
  MCU1_ControlTemp_S/1 -> MCU1_ControlTempcv/1
  MCU1_ControlTempcv/1 -> MCU1_ControlTemp_F/1
  MCU1_MotorTemp_F/1 -> MCU1_MotorTemp_Ad/1
  MCU1_MotorTemp_O/1 -> MCU1_MotorTemp_Ad/2
  MCU1_MotorTemp_Ad/1 -> MCU1_MotorTemp_sat/1
  MCU1_MotorTemp_sat/1 -> MCU1_MotorTemp_Out/1
  Demux/7 -> MCU1_MotorTemp_Sub/1(In1)
  MCU1_MotorTemp_Sub/1(Out1) -> MCU1_MotorTemp_Convert/1
  MCU1_MotorTemp_Convert/1 -> MCU1_MotorTemp_L/1
  MCU1_MotorTemp_L/1 -> MCU1_MotorTemp_S/1
  MCU1_MotorTemp_S/1 -> MCU1_MotorTempcv/1
  MCU1_MotorTempcv/1 -> MCU1_MotorTemp_F/1
  MCU1_PowerFdk_F/1 -> MCU1_PowerFdk_Ad/1
  MCU1_PowerFdk_O/1 -> MCU1_PowerFdk_Ad/2
  MCU1_PowerFdk_Ad/1 -> MCU1_PowerFdk_sat/1
  MCU1_PowerFdk_sat/1 -> MCU1_PowerFdk_Out/1
  Demux/5 -> MCU1_PowerFdkinput5_P/1
  MCU1_PowerFdkinput5_C/1 -> MCU1_PowerFdkinput5_P/2
  MCU1_PowerFdkinput5_P/1 -> MCU1_PowerFdkinput5_Ad/1
  Demux/6 -> MCU1_PowerFdkinput5_Ad/2
  MCU1_PowerFdkinput5_Ad/1 -> MCU1_PowerFdk_Sub/1(In1)
  MCU1_PowerFdk_Sub/1(Out1) -> MCU1_PowerFdk_Convert/1
  MCU1_PowerFdk_Convert/1 -> MCU1_PowerFdk_L/1
  MCU1_PowerFdk_L/1 -> MCU1_PowerFdk_S/1
  MCU1_PowerFdk_S/1 -> MCU1_PowerFdkcv/1
  MCU1_PowerFdkcv/1 -> MCU1_PowerFdk_F/1
  MCU1_Idc_F/1 -> MCU1_Idc_Ad/1
  MCU1_Idc_O/1 -> MCU1_Idc_Ad/2
  MCU1_Idc_Ad/1 -> MCU1_Idc_sat/1
  MCU1_Idc_sat/1 -> MCU1_Idc_Out/1
  Demux/3 -> MCU1_Idcinput3_P/1
  MCU1_Idcinput3_C/1 -> MCU1_Idcinput3_P/2
  MCU1_Idcinput3_P/1 -> MCU1_Idcinput3_Ad/1
  Demux/4 -> MCU1_Idcinput3_Ad/2
  MCU1_Idcinput3_Ad/1 -> MCU1_Idc_Sub/1(In1)
  MCU1_Idc_Sub/1(Out1) -> MCU1_Idc_Convert/1
  MCU1_Idc_Convert/1 -> MCU1_Idc_L/1
  MCU1_Idc_L/1 -> MCU1_Idc_S/1
  MCU1_Idc_S/1 -> MCU1_Idccv/1
  MCU1_Idccv/1 -> MCU1_Idc_F/1
  MCU1_Udc_F/1 -> MCU1_Udc_Ad/1
  MCU1_Udc_O/1 -> MCU1_Udc_Ad/2
  MCU1_Udc_Ad/1 -> MCU1_Udc_sat/1
  MCU1_Udc_sat/1 -> MCU1_Udc_Out/1
  Demux/1 -> MCU1_Udcinput1_P/1
  MCU1_Udcinput1_C/1 -> MCU1_Udcinput1_P/2
  MCU1_Udcinput1_P/1 -> MCU1_Udcinput1_Ad/1
  Demux/2 -> MCU1_Udcinput1_Ad/2
  MCU1_Udcinput1_Ad/1 -> MCU1_Udc_Sub/1(In1)
  MCU1_Udc_Sub/1(Out1) -> MCU1_Udc_Convert/1
  MCU1_Udc_Convert/1 -> MCU1_Udc_L/1
  MCU1_Udc_L/1 -> MCU1_Udc_S/1
  MCU1_Udc_S/1 -> MCU1_Udccv/1
  MCU1_Udccv/1 -> MCU1_Udc_F/1
  input/1 -> Demux/1

== system six_plus_six_AcmsteeringV09_main_1lf/Data_input/MCU1_4/MCU1 ==
  input : Inport
  Enable : EnablePort
  Demux : Demux  Outputs=8
  MCU1_ControlTemp_Ad : Sum
  MCU1_ControlTemp_Convert : DataTypeConversion  OutDataTypeStr=uint32
  MCU1_ControlTemp_F : Gain
  MCU1_ControlTemp_L : simulink/Logic and Bit Operations/Bitwise Operator  logicop=AND  UseBitMask=on  BitMask=255  BitMaskRealWorld=Stored Integer
  MCU1_ControlTemp_O : Constant  Value=-40  OutDataTypeStr=single
  MCU1_ControlTemp_S : ArithShift
  MCU1_ControlTemp_Sub : Subsystem
  MCU1_ControlTemp_sat : Saturate  UpperLimit=215  LowerLimit=-40
  MCU1_ControlTempcv : DataTypeConversion
  MCU1_Idc_Ad : Sum
  MCU1_Idc_Convert : DataTypeConversion  OutDataTypeStr=uint32
  MCU1_Idc_F : Gain  Gain=0.1
  MCU1_Idc_L : simulink/Logic and Bit Operations/Bitwise Operator  logicop=AND  UseBitMask=on  BitMask=65535  BitMaskRealWorld=Stored Integer
  MCU1_Idc_O : Constant  Value=-1600  OutDataTypeStr=single
  MCU1_Idc_S : ArithShift
  MCU1_Idc_Sub : Subsystem
  MCU1_Idc_sat : Saturate  UpperLimit=1600  LowerLimit=-1600
  MCU1_Idccv : DataTypeConversion
  MCU1_Idcinput3_Ad : Sum
  MCU1_Idcinput3_C : Constant  Value=256
  MCU1_Idcinput3_P : Product
  MCU1_MotorTemp_Ad : Sum
  MCU1_MotorTemp_Convert : DataTypeConversion  OutDataTypeStr=uint32
  MCU1_MotorTemp_F : Gain
  MCU1_MotorTemp_L : simulink/Logic and Bit Operations/Bitwise Operator  logicop=AND  UseBitMask=on  BitMask=255  BitMaskRealWorld=Stored Integer
  MCU1_MotorTemp_O : Constant  Value=-40  OutDataTypeStr=single
  MCU1_MotorTemp_S : ArithShift
  MCU1_MotorTemp_Sub : Subsystem
  MCU1_MotorTemp_sat : Saturate  UpperLimit=215  LowerLimit=-40
  MCU1_MotorTempcv : DataTypeConversion
  MCU1_PowerFdk_Ad : Sum
  MCU1_PowerFdk_Convert : DataTypeConversion  OutDataTypeStr=uint32
  MCU1_PowerFdk_F : Gain
  MCU1_PowerFdk_L : simulink/Logic and Bit Operations/Bitwise Operator  logicop=AND  UseBitMask=on  BitMask=65535  BitMaskRealWorld=Stored Integer
  MCU1_PowerFdk_O : Constant  Value=0  OutDataTypeStr=single
  MCU1_PowerFdk_S : ArithShift
  MCU1_PowerFdk_Sub : Subsystem
  MCU1_PowerFdk_sat : Saturate  UpperLimit=65535  LowerLimit=0
  MCU1_PowerFdkcv : DataTypeConversion
  MCU1_PowerFdkinput5_Ad : Sum
  MCU1_PowerFdkinput5_C : Constant  Value=256
  MCU1_PowerFdkinput5_P : Product
  MCU1_Udc_Ad : Sum
  MCU1_Udc_Convert : DataTypeConversion  OutDataTypeStr=uint32
  MCU1_Udc_F : Gain  Gain=0.1
  MCU1_Udc_L : simulink/Logic and Bit Operations/Bitwise Operator  logicop=AND  UseBitMask=on  BitMask=65535  BitMaskRealWorld=Stored Integer
  MCU1_Udc_O : Constant  Value=0  OutDataTypeStr=single
  MCU1_Udc_S : ArithShift
  MCU1_Udc_Sub : Subsystem
  MCU1_Udc_sat : Saturate  UpperLimit=1000  LowerLimit=0
  MCU1_Udccv : DataTypeConversion
  MCU1_Udcinput1_Ad : Sum
  MCU1_Udcinput1_C : Constant  Value=256
  MCU1_Udcinput1_P : Product
  MCU1_ControlTemp_Out : Outport
  MCU1_MotorTemp_Out : Outport  Port=2
  MCU1_PowerFdk_Out : Outport  Port=3
  MCU1_Idc_Out : Outport  Port=4
  MCU1_Udc_Out : Outport  Port=5
  wires:
  MCU1_ControlTemp_F/1 -> MCU1_ControlTemp_Ad/1
  MCU1_ControlTemp_O/1 -> MCU1_ControlTemp_Ad/2
  MCU1_ControlTemp_Ad/1 -> MCU1_ControlTemp_sat/1
  MCU1_ControlTemp_sat/1 -> MCU1_ControlTemp_Out/1
  Demux/8 -> MCU1_ControlTemp_Sub/1(In1)
  MCU1_ControlTemp_Sub/1(Out1) -> MCU1_ControlTemp_Convert/1
  MCU1_ControlTemp_Convert/1 -> MCU1_ControlTemp_L/1
  MCU1_ControlTemp_L/1 -> MCU1_ControlTemp_S/1
  MCU1_ControlTemp_S/1 -> MCU1_ControlTempcv/1
  MCU1_ControlTempcv/1 -> MCU1_ControlTemp_F/1
  MCU1_MotorTemp_F/1 -> MCU1_MotorTemp_Ad/1
  MCU1_MotorTemp_O/1 -> MCU1_MotorTemp_Ad/2
  MCU1_MotorTemp_Ad/1 -> MCU1_MotorTemp_sat/1
  MCU1_MotorTemp_sat/1 -> MCU1_MotorTemp_Out/1
  Demux/7 -> MCU1_MotorTemp_Sub/1(In1)
  MCU1_MotorTemp_Sub/1(Out1) -> MCU1_MotorTemp_Convert/1
  MCU1_MotorTemp_Convert/1 -> MCU1_MotorTemp_L/1
  MCU1_MotorTemp_L/1 -> MCU1_MotorTemp_S/1
  MCU1_MotorTemp_S/1 -> MCU1_MotorTempcv/1
  MCU1_MotorTempcv/1 -> MCU1_MotorTemp_F/1
  MCU1_PowerFdk_F/1 -> MCU1_PowerFdk_Ad/1
  MCU1_PowerFdk_O/1 -> MCU1_PowerFdk_Ad/2
  MCU1_PowerFdk_Ad/1 -> MCU1_PowerFdk_sat/1
  MCU1_PowerFdk_sat/1 -> MCU1_PowerFdk_Out/1
  Demux/5 -> MCU1_PowerFdkinput5_P/1
  MCU1_PowerFdkinput5_C/1 -> MCU1_PowerFdkinput5_P/2
  MCU1_PowerFdkinput5_P/1 -> MCU1_PowerFdkinput5_Ad/1
  Demux/6 -> MCU1_PowerFdkinput5_Ad/2
  MCU1_PowerFdkinput5_Ad/1 -> MCU1_PowerFdk_Sub/1(In1)
  MCU1_PowerFdk_Sub/1(Out1) -> MCU1_PowerFdk_Convert/1
  MCU1_PowerFdk_Convert/1 -> MCU1_PowerFdk_L/1
  MCU1_PowerFdk_L/1 -> MCU1_PowerFdk_S/1
  MCU1_PowerFdk_S/1 -> MCU1_PowerFdkcv/1
  MCU1_PowerFdkcv/1 -> MCU1_PowerFdk_F/1
  MCU1_Idc_F/1 -> MCU1_Idc_Ad/1
  MCU1_Idc_O/1 -> MCU1_Idc_Ad/2
  MCU1_Idc_Ad/1 -> MCU1_Idc_sat/1
  MCU1_Idc_sat/1 -> MCU1_Idc_Out/1
  Demux/3 -> MCU1_Idcinput3_P/1
  MCU1_Idcinput3_C/1 -> MCU1_Idcinput3_P/2
  MCU1_Idcinput3_P/1 -> MCU1_Idcinput3_Ad/1
  Demux/4 -> MCU1_Idcinput3_Ad/2
  MCU1_Idcinput3_Ad/1 -> MCU1_Idc_Sub/1(In1)
  MCU1_Idc_Sub/1(Out1) -> MCU1_Idc_Convert/1
  MCU1_Idc_Convert/1 -> MCU1_Idc_L/1
  MCU1_Idc_L/1 -> MCU1_Idc_S/1
  MCU1_Idc_S/1 -> MCU1_Idccv/1
  MCU1_Idccv/1 -> MCU1_Idc_F/1
  MCU1_Udc_F/1 -> MCU1_Udc_Ad/1
  MCU1_Udc_O/1 -> MCU1_Udc_Ad/2
  MCU1_Udc_Ad/1 -> MCU1_Udc_sat/1
  MCU1_Udc_sat/1 -> MCU1_Udc_Out/1
  Demux/1 -> MCU1_Udcinput1_P/1
  MCU1_Udcinput1_C/1 -> MCU1_Udcinput1_P/2
  MCU1_Udcinput1_P/1 -> MCU1_Udcinput1_Ad/1
  Demux/2 -> MCU1_Udcinput1_Ad/2
  MCU1_Udcinput1_Ad/1 -> MCU1_Udc_Sub/1(In1)
  MCU1_Udc_Sub/1(Out1) -> MCU1_Udc_Convert/1
  MCU1_Udc_Convert/1 -> MCU1_Udc_L/1
  MCU1_Udc_L/1 -> MCU1_Udc_S/1
  MCU1_Udc_S/1 -> MCU1_Udccv/1
  MCU1_Udccv/1 -> MCU1_Udc_F/1
  input/1 -> Demux/1
